simulink model "Add_Two_Numbers"  (R2022b)
settings: Solver=VariableStepAuto  StartTime=0.0  StopTime=10.0  RelTol=1e-3
libraries: simulink x1
settings Model: Creator=MAAM  LastModifiedBy=MAAM

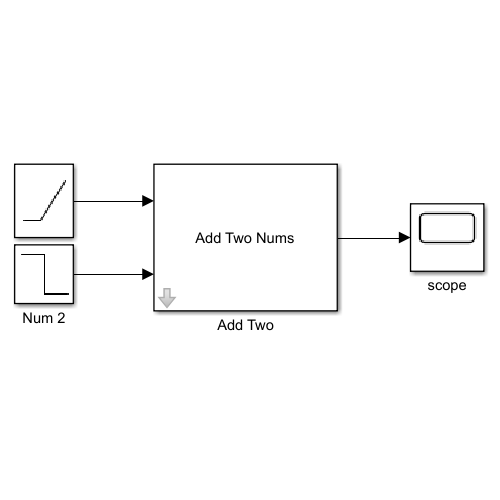
[thumbnail: Simulink's stored preview of the top-level diagram]
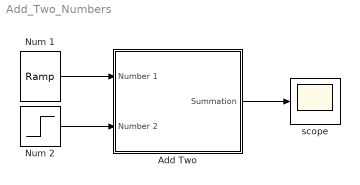
== system Add_Two_Numbers ==
  Add Two : Subsystem  mask(AddTwoNumbersSubSystemBlock){}
      mask help: SubSystem To add two numbers
      mask Display: disp("Add Two Nums")
  Num 1 : simulink/Sources/Ramp  slope=1  start=0  InitialOutput=0
  Num 2 : Step  Before=5  After=0  SampleTime=5
  scope : Scope
  wires:
  Num 1/1 -> Add Two/1(Number 1)
  Num 2/1 -> Add Two/2(Number 2)
  Add Two/1(Summation) -> scope/1

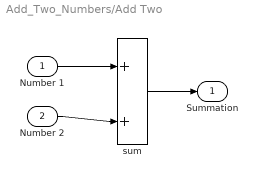
== system Add_Two_Numbers/Add Two ==
  Number 1 : Inport
  Number 2 : Inport  Port=2
  sum : Sum
  Summation : Outport
  wires:
  Number 1/1 -> sum/1
  Number 2/1 -> sum/2
  sum/1 -> Summation/1
